simulink library "INT_StSys_StrtRmp"  (R2016b)
settings: Solver=VariableStepAuto  StartTime=0.0  StopTime=10.0  RelTol=1e-3
settings Model: Creator=Administrator  LastModifiedBy=Administrator

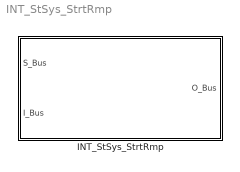
== system INT_StSys_StrtRmp ==
  INT_StSys_StrtRmp : Subsystem

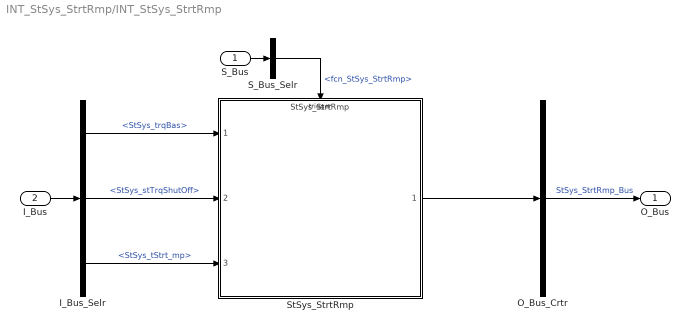
== system INT_StSys_StrtRmp/INT_StSys_StrtRmp ==
  S_Bus : Inport
  I_Bus : Inport  Port=2
  I_Bus_Selr : BusSelector  OutputSignals=StSys_trqBas,StSys_stTrqShutOff,StSys_tStrt_mp
  O_Bus_Crtr : BusCreator  Inputs=1
  S_Bus_Selr : BusSelector  OutputSignals=fcn_StSys_StrtRmp
  StSys_StrtRmp : ModelReference  ModelNameDialog=StSys_StrtRmp  SimulationMode=Normal  ModelReferenceVersion=1.51  TriggerPortName=function  TriggerPortTriggerType=function-call  TriggerPortStatesWhenEnabling=held
  O_Bus : Outport
  wires:
  S_Bus_Selr/1 -> StSys_StrtRmp/Trigger  "<fcn_StSys_StrtRmp>"
  S_Bus/1 -> S_Bus_Selr/1
  I_Bus/1 -> I_Bus_Selr/1
  I_Bus_Selr/1 -> StSys_StrtRmp/1  "<StSys_trqBas>"
  I_Bus_Selr/2 -> StSys_StrtRmp/2  "<StSys_stTrqShutOff>"
  I_Bus_Selr/3 -> StSys_StrtRmp/3  "<StSys_tStrt_mp>"
  O_Bus_Crtr/1 -> O_Bus/1  "StSys_StrtRmp_Bus"
  StSys_StrtRmp/1 -> O_Bus_Crtr/1
